simulink model "gm_uz_JL_SDDemodulator"  (R2025a)
settings: Solver=FixedStepDiscrete  StartTime=0.0  StopTime=0.001  RelTol=1e-3
undefined symbols (not defined in the file or in its folder): DiscIntNeverNeededParam
libraries: simulink x1, hdlsllib x1
settings Model: SimulationMode=accelerator  Creator=jonat  LastModifiedBy=jonat
settings SolverCC: AlgebraicLoopSolver=TrustRegion
settings DataIOCC: LimitDataPoints=on  SaveOutput=off  SaveTime=off
settings OptimizationCC: BlockReduction=off  ConditionallyExecuteInputs=off  DefaultParameterBehavior=Inlined  LifeSpan=inf
settings DebuggingCC: AlgebraicLoopMsg=error  InheritedTsInSrcMsg=none  SingleTaskRateTransMsg=error  UnconnectedInputMsg=warning  UnconnectedOutputMsg=warning  UnconnectedLineMsg=warning  AllowSymbolicDim=off  StrictBusMsg=ErrorOnBusTreatedAsVector  SFUnexpectedBacktrackingDiag=warning  SFNoUnconditionalDefaultTransitionDiag=warning  SFExecutionAtInitializationDiag=none  ArithmeticOperatorsInVariantConditions=warning
settings HardwareCC: ProdBitPerPointer=32.0  ProdBitPerSizeT=32.0  ProdBitPerPtrDiffT=32.0  ProdLargestAtomicFloat=None  ProdIntDivRoundTo=Undefined  ProdEndianess=Unspecified  ProdWordSize=32.0  ProdHWDeviceType=ASIC/FPGA->ASIC/FPGA  ProdEqTarget=off
settings ModelReferenceCC: EnableRefExpFcnMdlSchedulingChecks=on
settings SFSimCC: SimUseLocalCustomCode=off  CustomCodeUndefinedFunction=UseInterfaceOnly
settings RTWCC: RTWUseLocalCustomCode=off  GPUComputeCapability=3.5
settings CodeAppCC: StateflowObjectComments=on
settings GRTTargetCC: TargetLangStandard=C89/C90 (ANSI)
settings ConfigComp: CovScope=ReferencedModels  CovMetricSettings=dw  CovSaveCumulativeToWorkspaceVar=on  CovSaveSingleToWorkspaceVar=on  CovExternalEMLEnable=off  CovSFcnEnable=off

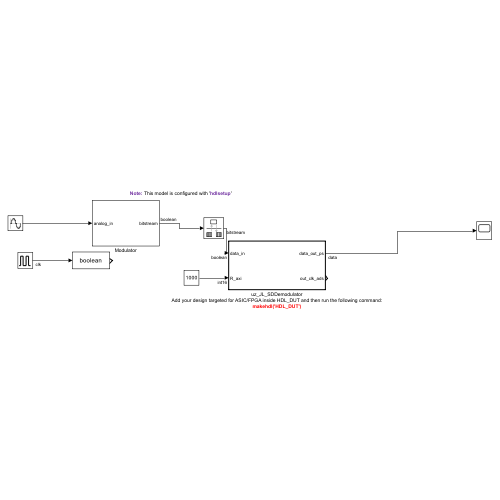
[thumbnail: Simulink's stored preview of the top-level diagram]
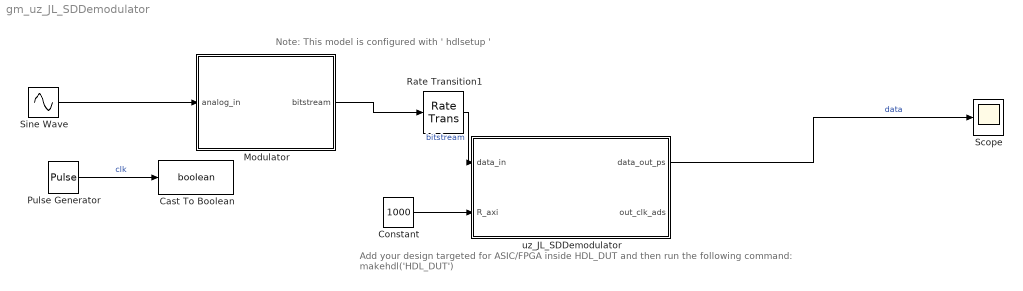
== system gm_uz_JL_SDDemodulator ==
  note: Add your design targeted for ASIC/FPGA inside HDL_DUT and then run the following command:
      | makehdl('HDL_DUT')
  note: Note: This model is configured with ' hdlsetup '
  Cast To Boolean : DataTypeConversion  OutDataTypeStr=boolean  SaturateOnIntegerOverflow=off  RndMeth=Floor
  Constant : Constant  Value=1000  OutDataTypeStr=int16
  Modulator : Subsystem
  Pulse Generator : DiscretePulseGenerator  PulseType=Time based  Period=1/10e6  PulseWidth=10
  Rate Transition1 : RateTransition
  Scope : Scope
      settings: ActiveDisplayYMinimum=-1.25E+8  ActiveDisplayYMaximum=1.25E+8
  Sine Wave : Sin  Amplitude=0.1  Frequency=2*pi*25  SampleTime=1e-7
  uz_JL_SDDemodulator : Subsystem  TreatAsAtomicUnit=on
  wires:
  uz_JL_SDDemodulator/1(data_out_ps) -> Scope/1  "data"
  Pulse Generator/1 -> Cast To Boolean/1  "clk"
  Rate Transition1/1 -> uz_JL_SDDemodulator/1(data_in)  "bitstream"
  Modulator/1(bitstream) -> Rate Transition1/1
  Sine Wave/1 -> Modulator/1(analog_in)
  Constant/1 -> uz_JL_SDDemodulator/2(R_axi)

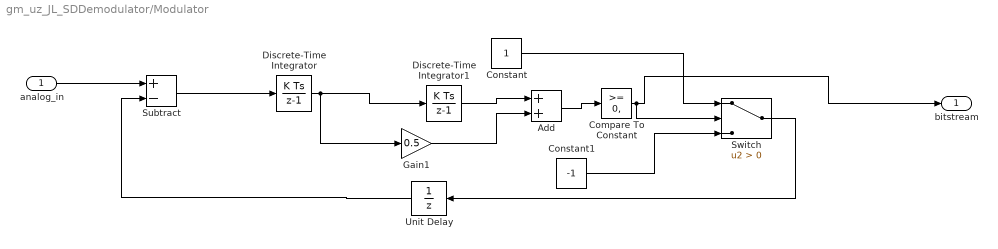
== system gm_uz_JL_SDDemodulator/Modulator ==
  analog_in : Inport
  Add : Sum
  Compare To Constant : simulink/Logic and Bit Operations/Compare To Constant  relop=>=  const=0,  OutDataTypeStr=boolean
  Constant : Constant
  Constant1 : Constant  Value=-1
  Discrete-Time Integrator : DiscreteIntegrator  SampleTime=1e-7  UpperSaturationLimit=2  LowerSaturationLimit=-2  ICPrevOutput=DiscIntNeverNeededParam  ICPrevScaledInput=DiscIntNeverNeededParam
  Discrete-Time Integrator1 : DiscreteIntegrator  SampleTime=1e-7  UpperSaturationLimit=2  LowerSaturationLimit=-2  ICPrevOutput=DiscIntNeverNeededParam  ICPrevScaledInput=DiscIntNeverNeededParam
  Gain1 : Gain  Gain=0.5
  Subtract : Sum  Inputs=+-  OutDataTypeStr=double
  Switch : Switch  Criteria=u2 > Threshold  OutDataTypeStr=fixdt(1,2,0)  SaturateOnIntegerOverflow=off  InputSameDT=off
  Unit Delay : UnitDelay  SampleTime=-1  HasFrameUpgradeWarning=on
  bitstream : Outport  OutDataTypeStr=boolean
  wires:
  Add/1 -> Compare To Constant/1
  Gain1/1 -> Add/2
  Unit Delay/1 -> Subtract/2
  Constant1/1 -> Switch/3
  Constant/1 -> Switch/1
  Compare To Constant/1 -> Switch/2, bitstream/1
  Switch/1 -> Unit Delay/1
  Subtract/1 -> Discrete-Time Integrator/1
  Discrete-Time Integrator1/1 -> Add/1
  Discrete-Time Integrator/1 -> Discrete-Time Integrator1/1, Gain1/1
  analog_in/1 -> Subtract/1

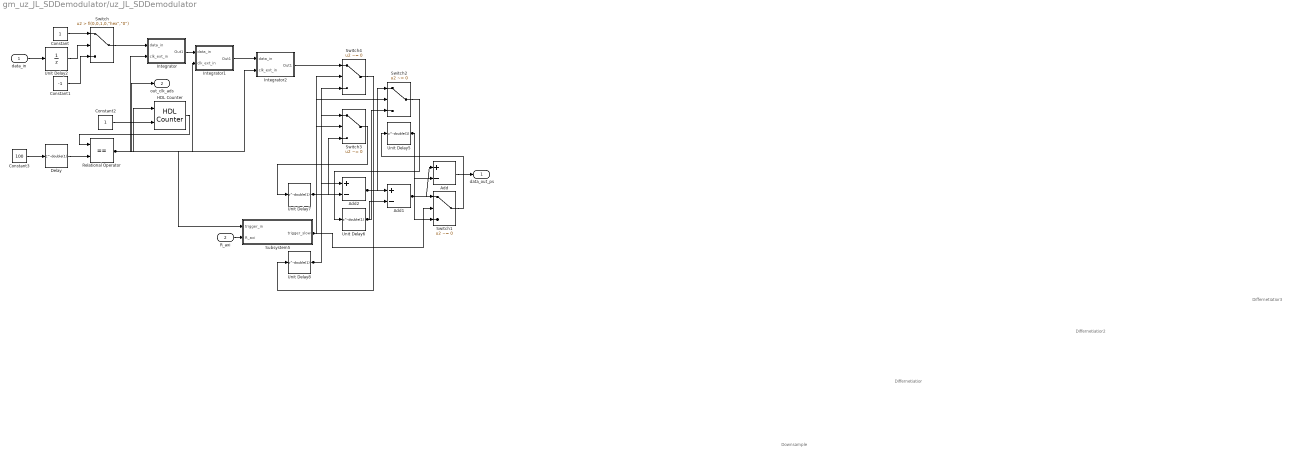
== system gm_uz_JL_SDDemodulator/uz_JL_SDDemodulator ==
  note: Differnetiatior3
  note: Differnetiatior2
  note: Differnetiatior
  note: Downsample
  data_in : Inport  OutDataTypeStr=boolean  PortDimensions=1  SampleTime=1e-08
  R_axi : Inport  Port=2  OutDataTypeStr=int16  PortDimensions=1  SampleTime=1e-08
  Add : Sum  Inputs=+-  OutDataTypeStr=int32  AccumDataTypeStr=int32  SampleTime=1e-08
  Add1 : Sum  Inputs=+-  OutDataTypeStr=int32  AccumDataTypeStr=int32  SampleTime=1e-08
  Add2 : Sum  Inputs=+-  OutDataTypeStr=int32  AccumDataTypeStr=int32  SampleTime=1e-08
  Constant : Constant  OutDataTypeStr=int32  SampleTime=1e-08
  Constant1 : Constant  Value=-1  OutDataTypeStr=int32  SampleTime=1e-08
  Constant2 : Constant  OutDataTypeStr=boolean  SampleTime=1e-08
  Constant3 : Constant  Value=100  OutDataTypeStr=uint8  SampleTime=1e-08
  Delay : Delay  DelayLength=double(1)  InitialCondition=0  SampleTime=1e-08
  HDL Counter : hdlsllib/Sources/HDL Counter  CountType=Free running  CountInit=0  CountStep=1  CountMax=25  CountFromType=Initial value  CountFrom=0  CountResetPort=on  CountLoadPort=off  CountEnbPort=on  CountDirPort=off  CountHitOutputPort=off  CountDataType=Unsigned  CountWordLen=8  CountFracLen=0  CountSampTime=1
  Integrator : Subsystem
  Integrator1 : Subsystem
  Integrator2 : Subsystem
  Relational Operator : RelationalOperator  Operator===  OutDataTypeStr=boolean  SampleTime=1e-08  InputSameDT=off
  Subsystem5 : Subsystem
  Switch : Switch  Criteria=u2 > Threshold  Threshold="fi(0,0,1,0,\"hex\",\"0\")"  OutDataTypeStr=int32  SampleTime=1e-08  SaturateOnIntegerOverflow=off  InputSameDT=off
  Switch{1..4} (4 alike) : Switch  Criteria=u2 ~= 0  Threshold="fi(0,0,1,0,\"hex\",\"0\")"  OutDataTypeStr=int32  SampleTime=1e-08  SaturateOnIntegerOverflow=off  InputSameDT=off
  Unit Delay2 : UnitDelay  SampleTime=1e-08
  Unit Delay{5..8} (4 alike) : Delay  DelayLength=double(1)  InitialCondition=0  SampleTime=1e-08
  data_out_ps : Outport  SampleTime=1e-08
  out_clk_ads : Outport  Port=2  SampleTime=1e-08
  wires:
  data_in/1 -> Unit Delay2/1
  Delay/1 -> Relational Operator/2
  Constant2/1 -> HDL Counter/2
  Unit Delay6/1 -> Switch2/3, Add1/2
  Constant1/1 -> Switch/3
  Unit Delay2/1 -> Switch/2
  Constant/1 -> Switch/1
  Constant3/1 -> Delay/1
  Switch/1 -> Integrator/1(data_in)
  Relational Operator/1 -> Integrator2/2(clk_ext_in), Integrator1/2(clk_ext_in), Subsystem5/1(trigger_in), Integrator/2(clk_ext_in), out_clk_ads/1, HDL Counter/1
  Unit Delay5/1 -> Switch1/3, Add/2
  Subsystem5/1(trigger_slow) -> Switch2/2, Switch4/2, Switch3/2, Switch1/2
  Integrator/1(Out1) -> Integrator1/1(data_in)
  HDL Counter/1 -> Relational Operator/1
  Add1/1 -> Add/1, Switch1/1
  R_axi/1 -> Subsystem5/2(R_axi)
  Integrator1/1(Out1) -> Integrator2/1(data_in)
  Unit Delay8/1 -> Switch4/3, Switch3/1, Add2/1
  Integrator2/1(Out1) -> Switch4/1
  Unit Delay7/1 -> Switch3/3, Add2/2
  Switch4/1 -> Unit Delay8/1
  Add/1 -> data_out_ps/1
  Switch3/1 -> Unit Delay7/1
  Add2/1 -> Switch2/1, Add1/1
  Switch2/1 -> Unit Delay6/1
  Switch1/1 -> Unit Delay5/1

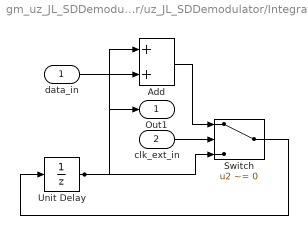
== system gm_uz_JL_SDDemodulator/uz_JL_SDDemodulator/Integrator ==
  data_in : Inport  OutDataTypeStr=int32  PortDimensions=1  SampleTime=1e-08
  clk_ext_in : Inport  Port=2  OutDataTypeStr=boolean  PortDimensions=1  SampleTime=1e-08
  Add : Sum  OutDataTypeStr=int32
  Switch : Switch  Criteria=u2 ~= 0  OutDataTypeStr=int32  SaturateOnIntegerOverflow=off  InputSameDT=off
  Unit Delay : UnitDelay  SampleTime=1e-8  HasFrameUpgradeWarning=on
  Out1 : Outport  SampleTime=1e-08
  wires:
  clk_ext_in/1 -> Switch/2
  Add/1 -> Switch/1
  Unit Delay/1 -> Switch/3, Add/1, Out1/1
  data_in/1 -> Add/2
  Switch/1 -> Unit Delay/1

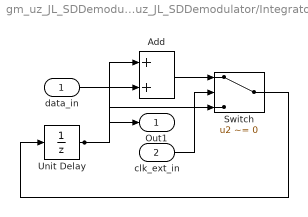
== system gm_uz_JL_SDDemodulator/uz_JL_SDDemodulator/Integrator1 ==
  data_in : Inport  OutDataTypeStr=int32  PortDimensions=1  SampleTime=1e-08
  clk_ext_in : Inport  Port=2  OutDataTypeStr=boolean  PortDimensions=1  SampleTime=1e-08
  Add : Sum  OutDataTypeStr=fixdt(1,32,0)  AccumDataTypeStr=fixdt(1,32,0)
  Switch : Switch  Criteria=u2 ~= 0  OutDataTypeStr=fixdt(1,32,0)  SaturateOnIntegerOverflow=off  InputSameDT=off
  Unit Delay : UnitDelay  SampleTime=1e-8  HasFrameUpgradeWarning=on
  Out1 : Outport  SampleTime=1e-08
  wires:
  data_in/1 -> Add/2
  Add/1 -> Switch/1
  Unit Delay/1 -> Switch/3, Add/1, Out1/1
  clk_ext_in/1 -> Switch/2
  Switch/1 -> Unit Delay/1

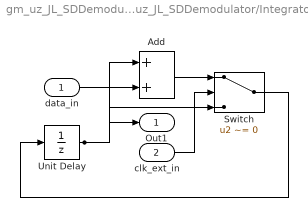
== system gm_uz_JL_SDDemodulator/uz_JL_SDDemodulator/Integrator2 ==
  data_in : Inport  OutDataTypeStr=int32  PortDimensions=1  SampleTime=1e-08
  clk_ext_in : Inport  Port=2  OutDataTypeStr=boolean  PortDimensions=1  SampleTime=1e-08
  Add : Sum  OutDataTypeStr=fixdt(1,32,0)  AccumDataTypeStr=fixdt(1,32,0)
  Switch : Switch  Criteria=u2 ~= 0  OutDataTypeStr=fixdt(1,32,0)  SaturateOnIntegerOverflow=off  InputSameDT=off
  Unit Delay : UnitDelay  SampleTime=1e-8  HasFrameUpgradeWarning=on
  Out1 : Outport  SampleTime=1e-08
  wires:
  clk_ext_in/1 -> Switch/2
  Add/1 -> Switch/1
  data_in/1 -> Add/2
  Unit Delay/1 -> Switch/3, Add/1, Out1/1
  Switch/1 -> Unit Delay/1

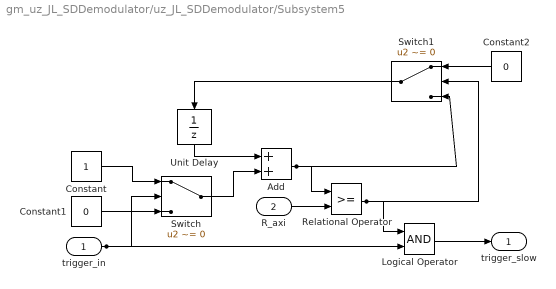
== system gm_uz_JL_SDDemodulator/uz_JL_SDDemodulator/Subsystem5 ==
  trigger_in : Inport  OutDataTypeStr=boolean  PortDimensions=1  SampleTime=1e-08
  R_axi : Inport  Port=2  OutDataTypeStr=int16  PortDimensions=1  SampleTime=1e-08
  Add : Sum  OutDataTypeStr=fixdt(1,32,0)
  Constant : Constant  OutDataTypeStr=fixdt(1,32,0)  SampleTime=-1
  Constant1 : Constant  Value=0  OutDataTypeStr=fixdt(1,32,0)  SampleTime=-1
  Constant2 : Constant  Value=0  OutDataTypeStr=fixdt(1,32,0)  SampleTime=-1
  Logical Operator : Logic  AllPortsSameDT=off  OutDataTypeStr=boolean
  Relational Operator : RelationalOperator  OutDataTypeStr=boolean  RndMeth=Simplest  InputSameDT=off
  Switch : Switch  Criteria=u2 ~= 0  OutDataTypeStr=fixdt(1,32,0)  SaturateOnIntegerOverflow=off  InputSameDT=off
  Switch1 : Switch  Criteria=u2 ~= 0  OutDataTypeStr=fixdt(1,32,0)  SaturateOnIntegerOverflow=off  InputSameDT=off
  Unit Delay : UnitDelay  SampleTime=-1  HasFrameUpgradeWarning=on
  trigger_slow : Outport  SampleTime=1e-08
  wires:
  Switch/1 -> Add/2
  Unit Delay/1 -> Add/1
  Constant/1 -> Switch/1
  R_axi/1 -> Relational Operator/2
  Constant1/1 -> Switch/3
  trigger_in/1 -> Logical Operator/2, Switch/2
  Add/1 -> Switch1/3, Relational Operator/1
  Relational Operator/1 -> Switch1/2, Logical Operator/1
  Switch1/1 -> Unit Delay/1
  Logical Operator/1 -> trigger_slow/1
  Constant2/1 -> Switch1/1
